simulink model "sl_subsys_fcncallerr13"  (Simulink 7.6)
settings: Solver=FixedStepDiscrete  StartTime=0.0  StopTime=10.0  RelTol=1e-3
libraries: simulink x5
settings Model: Creator=The MathWorks Inc.
settings DataIOCC: SaveState=on
settings DebuggingCC: UnderspecifiedInitializationDetection=Simplified  StrictBusMsg=ErrorOnBusTreatedAsVector
settings SFSimCC: SimParseCustomCode=off

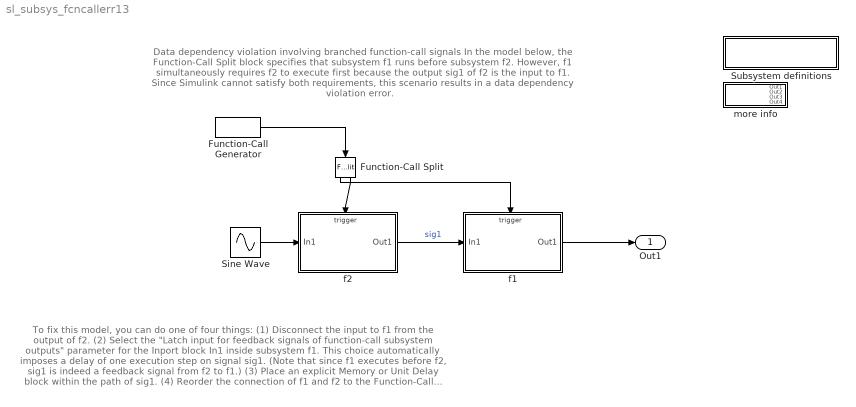
== system sl_subsys_fcncallerr13 ==
  note: To fix this model, you can do one of four things:
      | (1) Disconnect the input to f1 from the output of f2.
      | (2) Select the "Latch input for feedback signals of function-call subsystem outputs"
      |     parameter for the Inport block In1 inside subsystem f1. This choice automatically
      |     imposes a delay of one execution step on signal sig1. (Note that since f1 executes
      |     before f2, sig1 is indeed a feedback signal from f2 to f1.)
      | (3) Place an explicit Memory or Unit Delay block within the path of sig1.
      | (4) Reorder the connection of f1 and f2 to the Function-Call Split block.
  note: Data dependency violation involving branched function-call signals
      |
      | In the model below, the Function-Call Split block specifies that
      | subsystem f1 runs before subsystem f2. However, f1 simultaneously
      | requires f2 to execute first because the output sig1 of f2 is the input
      | to f1. Since Simulink cannot satisfy both requirements, this scenario
      | results in a data dependency violation error.
  " Subsystem definitions" : Subsystem
      settings: OpenFcn=helpview([matlabroot,'/toolbox/simulink/simdemos/simfeatures/html/sl_subsys_definitions.html']);
      mask Display: disp('Subsystem\ndefinitions')
  Function-Call Generator : simulink/Ports & Subsystems/Function-Call Generator  sample_time=1  numberOfIterations=1
  Function-Call Split : FunctionCallSplit
  Sine Wave : Sin  SampleTime=1
  f1 : Subsystem  TreatAsAtomicUnit=on
  f2 : Subsystem  TreatAsAtomicUnit=on
  more info : Subsystem
      mask Display: disp(get_param(gcb,'name'))
  Out1 : Outport
  wires:
  Function-Call Generator/1 -> Function-Call Split/1
  f1/1(Out1) -> Out1/1
  Sine Wave/1 -> f2/1(In1)
  Function-Call Split/2 -> f2/Trigger
  Function-Call Split/1 -> f1/Trigger
  f2/1(Out1) -> f1/1(In1)  "sig1"

== system sl_subsys_fcncallerr13/ Subsystem definitions ==

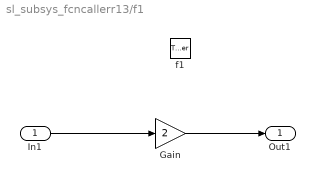
== system sl_subsys_fcncallerr13/f1 ==
  In1 : Inport
  f1 : TriggerPort  TriggerType=function-call  SampleTimeType=periodic
  Gain : Gain  Gain=2
  Out1 : Outport  InitialOutput=1/1000
      settings: AttributesFormatString=%<OutputWhenDisabled>: %<InitialOutput>
  wires:
  Gain/1 -> Out1/1
  In1/1 -> Gain/1

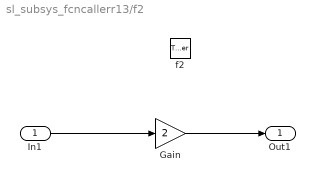
== system sl_subsys_fcncallerr13/f2 ==
  In1 : Inport
  f2 : TriggerPort  TriggerType=function-call  SampleTimeType=periodic
  Gain : Gain  Gain=2
  Out1 : Outport  InitialOutput=1/1000
      settings: AttributesFormatString=%<OutputWhenDisabled>: %<InitialOutput>
  wires:
  In1/1 -> Gain/1
  Gain/1 -> Out1/1

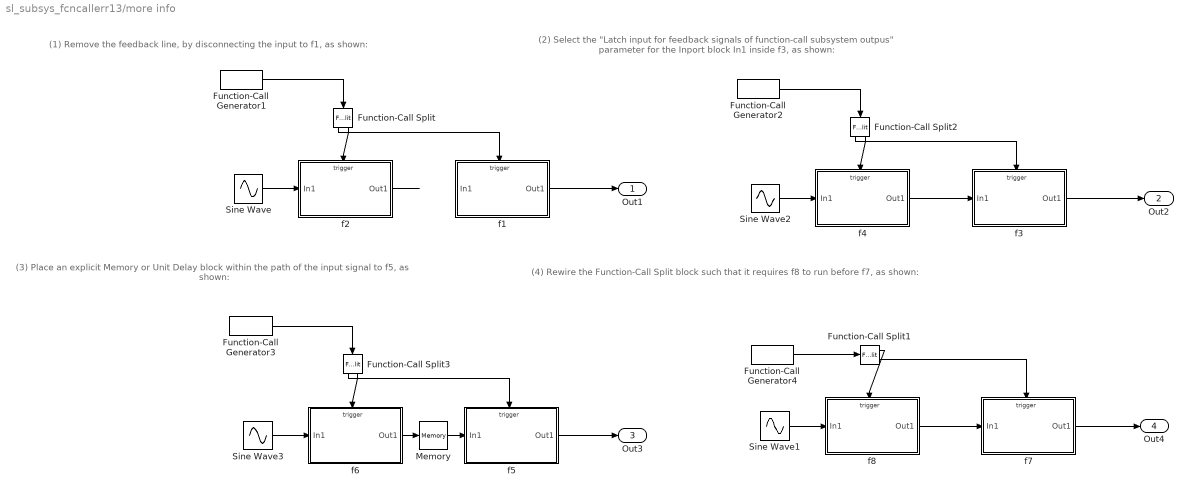
== system sl_subsys_fcncallerr13/more info ==
  note: (1) Remove the feedback line, by disconnecting the input to f1, as shown:
  note: (2) Select the "Latch input for feedback signals of function-call subsystem
      |     outpus" parameter for the Inport block In1 inside f3, as shown:
  note: (3) Place an explicit Memory or Unit Delay block within the path of the
      |     input signal to f5, as shown:
  note: (4) Rewire the Function-Call Split block such that it requires f8 to run
      |     before f7, as shown:
  Function-Call Generator{1..4} (4 alike) : simulink/Ports & Subsystems/Function-Call Generator  sample_time=1  numberOfIterations=1
  Function-Call Split{,1..3} (4 alike) : FunctionCallSplit
  Memory : Memory
  Sine Wave{,1..3} (4 alike) : Sin  SampleTime=1
  f1 : Subsystem  TreatAsAtomicUnit=on
  f2 : Subsystem  TreatAsAtomicUnit=on
  f3 : Subsystem  TreatAsAtomicUnit=on
  f4 : Subsystem  TreatAsAtomicUnit=on
  f5 : Subsystem  TreatAsAtomicUnit=on
  f6 : Subsystem  TreatAsAtomicUnit=on
  f7 : Subsystem  TreatAsAtomicUnit=on
  f8 : Subsystem  TreatAsAtomicUnit=on
  Out1 : Outport
  Out2 : Outport  Port=2
  Out3 : Outport  Port=3
  Out4 : Outport  Port=4
  wires:
  Function-Call Generator1/1 -> Function-Call Split/1
  f1/1(Out1) -> Out1/1
  Sine Wave/1 -> f2/1(In1)
  Function-Call Split/2 -> f2/Trigger
  Function-Call Split/1 -> f1/Trigger
  f2/1(Out1) -> ?
  Sine Wave1/1 -> f8/1(In1)
  f8/1(Out1) -> f7/1(In1)
  Function-Call Generator4/1 -> Function-Call Split1/1
  Function-Call Split1/1 -> f8/Trigger
  Function-Call Split1/2 -> f7/Trigger
  Function-Call Generator2/1 -> Function-Call Split2/1
  Sine Wave2/1 -> f4/1(In1)
  Function-Call Split2/2 -> f4/Trigger
  Function-Call Split2/1 -> f3/Trigger
  f4/1(Out1) -> f3/1(In1)
  Function-Call Generator3/1 -> Function-Call Split3/1
  Sine Wave3/1 -> f6/1(In1)
  Function-Call Split3/2 -> f6/Trigger
  Function-Call Split3/1 -> f5/Trigger
  f6/1(Out1) -> Memory/1
  Memory/1 -> f5/1(In1)
  f3/1(Out1) -> Out2/1
  f7/1(Out1) -> Out4/1
  f5/1(Out1) -> Out3/1

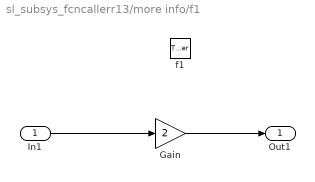
== system sl_subsys_fcncallerr13/more info/f1 ==
  In1 : Inport
  f1 : TriggerPort  TriggerType=function-call  SampleTimeType=periodic
  Gain : Gain  Gain=2
  Out1 : Outport  InitialOutput=1/1000
      settings: AttributesFormatString=%<OutputWhenDisabled>: %<InitialOutput>
  wires:
  In1/1 -> Gain/1
  Gain/1 -> Out1/1

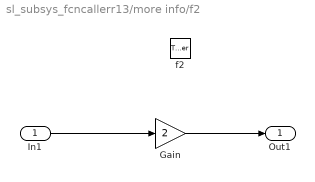
== system sl_subsys_fcncallerr13/more info/f2 ==
  In1 : Inport
  f2 : TriggerPort  TriggerType=function-call  SampleTimeType=periodic
  Gain : Gain  Gain=2
  Out1 : Outport  InitialOutput=1/1000
      settings: AttributesFormatString=%<OutputWhenDisabled>: %<InitialOutput>
  wires:
  Gain/1 -> Out1/1
  In1/1 -> Gain/1

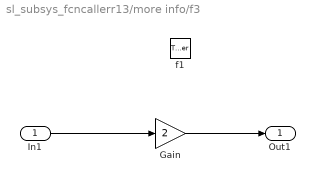
== system sl_subsys_fcncallerr13/more info/f3 ==
  In1 : Inport
      settings: LatchInputForFeedbackSignals=on
  f1 : TriggerPort  TriggerType=function-call  SampleTimeType=periodic
  Gain : Gain  Gain=2
  Out1 : Outport  InitialOutput=1/1000
      settings: AttributesFormatString=%<OutputWhenDisabled>: %<InitialOutput>
  wires:
  Gain/1 -> Out1/1
  In1/1 -> Gain/1

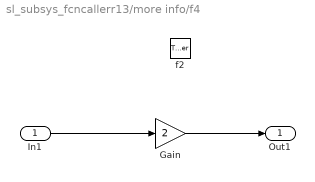
== system sl_subsys_fcncallerr13/more info/f4 ==
  In1 : Inport
  f2 : TriggerPort  TriggerType=function-call  SampleTimeType=periodic
  Gain : Gain  Gain=2
  Out1 : Outport  InitialOutput=1/1000
      settings: AttributesFormatString=%<OutputWhenDisabled>: %<InitialOutput>
  wires:
  In1/1 -> Gain/1
  Gain/1 -> Out1/1

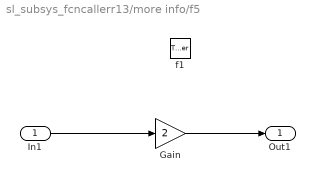
== system sl_subsys_fcncallerr13/more info/f5 ==
  In1 : Inport
      settings: LatchInputForFeedbackSignals=on
  f1 : TriggerPort  TriggerType=function-call  SampleTimeType=periodic
  Gain : Gain  Gain=2
  Out1 : Outport  InitialOutput=1/1000
      settings: AttributesFormatString=%<OutputWhenDisabled>: %<InitialOutput>
  wires:
  In1/1 -> Gain/1
  Gain/1 -> Out1/1

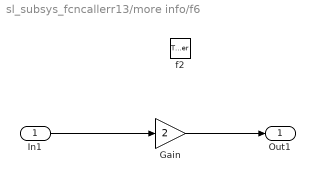
== system sl_subsys_fcncallerr13/more info/f6 ==
  In1 : Inport
  f2 : TriggerPort  TriggerType=function-call  SampleTimeType=periodic
  Gain : Gain  Gain=2
  Out1 : Outport  InitialOutput=1/1000
      settings: AttributesFormatString=%<OutputWhenDisabled>: %<InitialOutput>
  wires:
  Gain/1 -> Out1/1
  In1/1 -> Gain/1

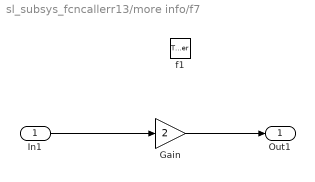
== system sl_subsys_fcncallerr13/more info/f7 ==
  In1 : Inport
  f1 : TriggerPort  TriggerType=function-call  SampleTimeType=periodic
  Gain : Gain  Gain=2
  Out1 : Outport  InitialOutput=1/1000
      settings: AttributesFormatString=%<OutputWhenDisabled>: %<InitialOutput>
  wires:
  Gain/1 -> Out1/1
  In1/1 -> Gain/1

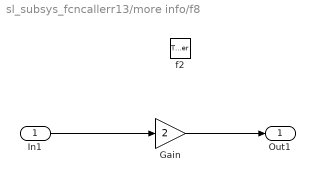
== system sl_subsys_fcncallerr13/more info/f8 ==
  In1 : Inport
  f2 : TriggerPort  TriggerType=function-call  SampleTimeType=periodic
  Gain : Gain  Gain=2
  Out1 : Outport  InitialOutput=1/1000
      settings: AttributesFormatString=%<OutputWhenDisabled>: %<InitialOutput>
  wires:
  In1/1 -> Gain/1
  Gain/1 -> Out1/1
